simulink model "control"  (R2022a)
settings: Solver=FixedStepAuto  StartTime=0.0  StopTime=Inf  FixedStep=Ts  RelTol=1e-3  EnableMultiTasking=on
undefined symbols (not defined in the file): Analog_max, Calib_Gain, GPTRIP1SEL, Ipeak, Ki_i, Kp_i, Kp_w, Kt, Offset, Ts, TZ1, V_AImax, Vbat, Vnom, w_motor_max
libraries: c2837xDlib x3, c2802xlib x3, slpidlib x2, c280xlib x2
settings Model: SimulationMode=external  ExtModeTrigDuration=8  Creator=34688  LastModifiedBy=manu.sanchez
settings SolverCC: AutoInsertRateTranBlk=on
settings OptimizationCC: DefaultUnderspecifiedDataType=single  EnhancedBackFolding=on  PassReuseOutputArgsAs=Individual arguments  MaxStackSize=1024  OptimizeBlockOrder=speed  DifferentSizesBufferReuse=on  OptimizationCustomize=off  DenormalBehavior=FlushToZero  EfficientTunableParamExpr=on
settings DebuggingCC: ParameterTunabilityLossMsg=error  UnconnectedInputMsg=warning  UnconnectedOutputMsg=warning  UnconnectedLineMsg=warning
settings HardwareCC: ProdBitPerChar=16  ProdBitPerInt=16  ProdBitPerPointer=32  ProdBitPerSizeT=32  ProdBitPerPtrDiffT=32  ProdLargestAtomicInteger=Integer  ProdLargestAtomicFloat=None  ProdWordSize=16  ProdLongLongMode=on  ProdHWDeviceType=Texas Instruments->C2000
settings SFSimCC: MATLABDynamicMemAlloc=off
settings RTWCC: SystemTargetFile=ert.tlc  HardwareBoard=TI Delfino F28379D LaunchPad  TemplateMakefile=ert_default_tmf  Toolchain=Texas Instruments Code Composer Studio (C2000)  DLArmComputeVersion=19.05
settings CodeAppCC: ForceParamTrailComments=on  IgnoreCustomStorageClasses=off  OperatorAnnotations=on  SimulinkDataObjDesc=on  SFDataObjDesc=on  InsertBlockDesc=on
settings ERTTargetCC: CodeReplacementLibrary=TI C28x  SupportContinuousTime=on  ExtModeTransport=3  ExtModeStaticAllocSize=10000

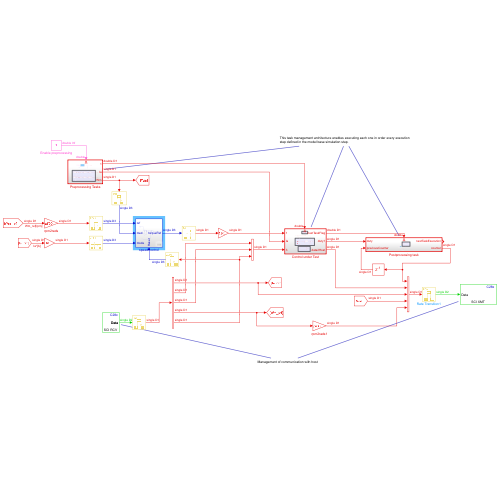
[thumbnail: Simulink's stored preview of the top-level diagram]
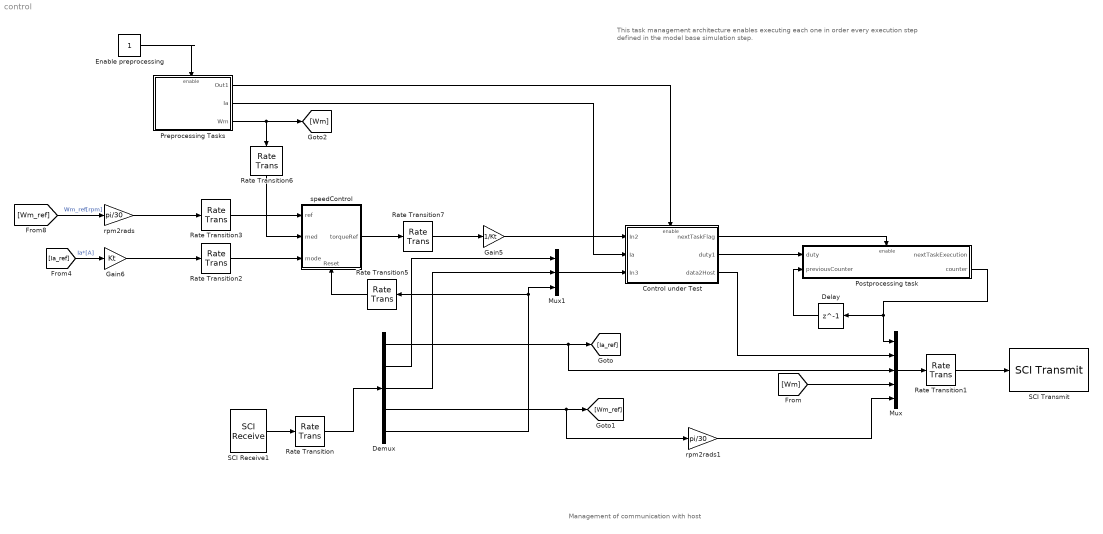
== system control ==
  note: This task management architecture enables executing each one in order every execution step defined in the model base simulation step.
  note: Management of communication with host
  Control under Test : Subsystem  TreatAsAtomicUnit=on
  Delay : Delay  DelayLength=1
  Demux : Demux  Outputs=5
  Enable preprocessing : Constant
  Gain5 : Gain  Gain=1/Kt
  Gain6 : Gain  Gain=Kt
  Mux : Mux  Inputs=5
  Mux1 : Mux  Inputs=3
  Postprocessing task : Subsystem  TreatAsAtomicUnit=on
  Preprocessing Tasks : Subsystem  TreatAsAtomicUnit=on
  Rate Transition : RateTransition  OutPortSampleTime=Ts
  Rate Transition1 : RateTransition  OutPortSampleTime=1e-3
  Rate Transition{2..3,5..6} (4 alike) : RateTransition  OutPortSampleTime=Ts*10
  Rate Transition7 : RateTransition  OutPortSampleTime=Ts
  SCI Receive1 : c280xlib/SCI Receive  sciModule=A  dataHead='S'  headerCheckMaxCount=16  dataTail='E'  dataType=single  dataLenOptions=Length via dialog  dataDim=5  maxDataLength=1  initValue=0  errOption=Output the last received value  errValue=0  sampleTime=0.001  blockingMode=on  timeOut=0.00875  outputStatus=off
      settings: SourceProductBaseCode=TIC2000
  SCI Transmit : c280xlib/SCI Transmit  sciModule=A  dataHead='S'  dataTail='E'  blockingMode=on  outputStatus=off
  rpm2rads : Gain  Gain=pi/30
  rpm2rads1 : Gain  Gain=pi/30
  speedControl : Subsystem
      settings: PortSchema="{\"entries\":[{\"content\":{\"sides\":[{\"content\":{\"connectorIds\":[\"In1\",\"In2\",\"In3\"]},\"type\":\"ConnectorPlacement.EquallySpacedRectSide\",\"uuid\":\"717e16ee-b0d7-408d-ae9c-739de9edb354\"},{\"content\":{\"connectorIds\":[\"Out1\"],\"side\":\"RIGHT\"},\"type\":\"ConnectorPlacement.EquallySpacedRectSide\",\"uuid\":\"4d51b045-d1f8-4970-b864-a989cb97e64e\"},{\"content\":{\"connectorIds\":[],\"side\":\"TOP\"},\"type\":\"ConnectorPlacement.EquallySpacedRectSide\",\"uuid\":\"4742e6f1-9767-49c3-9346-1403913518ce\"},{\"content\":{\"connectorIds\":[\"In4\"],\"side\":\"BOTTOM\"},\"type\":\"ConnectorPlacement.EquallySpacedRectSide\",\"uuid\":\"c526dc22-4687-4073-9922-de56cfbf6450\"}]},\"type\":\"ConnectorPlacement.EquallySpacedConnector\",\"uuid\":\"5f2e596d-c564-4cf7-8e3e-10d76f0f6b09\"}],\"packageUris\":[\"http://schema.mathworks.com/mf0/Connector/R2020b\"],\"version\":\"1.0\"}"
  wires:
  Control under Test/1(nextTaskFlag) -> Postprocessing task/Enable
  Enable preprocessing/1 -> Preprocessing Tasks/Enable
  SCI Receive1/1 -> Rate Transition/1
  Rate Transition1/1 -> SCI Transmit/1
  Control under Test/2(duty1) -> Postprocessing task/1(duty)
  Mux/1 -> Rate Transition1/1
  Control under Test/3(data2Host) -> Mux/2
  Postprocessing task/2(counter) -> Mux/1, Delay/1
  Delay/1 -> Postprocessing task/2(previousCounter)
  Preprocessing Tasks/1(Out1) -> Control under Test/Enable
  [Wm_ref] -> rpm2rads/1  "Wm_ref[rpm]"
  Gain6/1 -> Rate Transition2/1
  Preprocessing Tasks/3(Wm) -> Rate Transition6/1, [Wm]
  Demux/5 -> Rate Transition5/1, Mux1/3
  rpm2rads/1 -> Rate Transition3/1
  [Ia_ref] -> Gain6/1  "Ia*[A]"
  speedControl/1(torqueRef) -> Rate Transition7/1
  Rate Transition/1 -> Demux/1
  Demux/1 -> Mux/3, [Ia_ref]
  Demux/4 -> rpm2rads1/1, [Wm_ref]
  Mux1/1 -> Control under Test/3(In3)
  Demux/2 -> Mux1/1
  Demux/3 -> Mux1/2
  Preprocessing Tasks/2(Ia) -> Control under Test/2(Ia)
  Rate Transition2/1 -> speedControl/3(mode)
  Rate Transition3/1 -> speedControl/1(ref)
  Gain5/1 -> Control under Test/1(In2)
  Rate Transition5/1 -> speedControl/4(Reset)
  Rate Transition6/1 -> speedControl/2(med)
  Rate Transition7/1 -> Gain5/1
  [Wm] -> Mux/4
  rpm2rads1/1 -> Mux/5

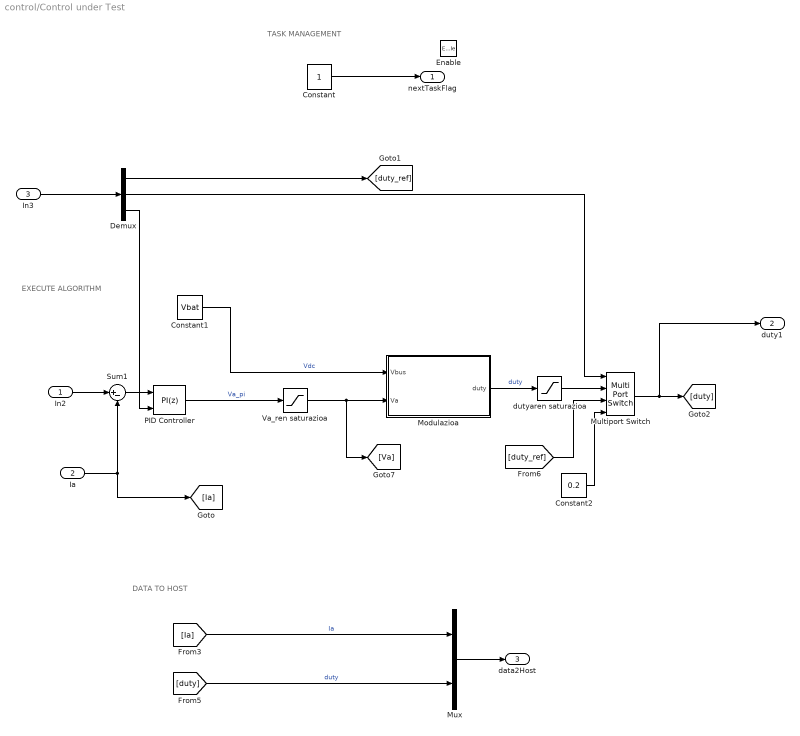
== system control/Control under Test ==
  note: TASK MANAGEMENT
  note: EXECUTE ALGORITHM
  note: DATA TO HOST
  In2 : Inport
  Ia : Inport  Port=2
  In3 : Inport  Port=3
  Enable : EnablePort
  Constant : Constant
  Constant1 : Constant  Value=Vbat  OutDataTypeStr=single
  Constant2 : Constant  Value=0.2  OutDataTypeStr=single  SampleTime=200e-6
  Demux : Demux  Outputs=3
  Modulazioa : Subsystem  Variant=on  VariantControlMode=label  LabelModeActiveChoice=MODULAZIOA_ZUBI_ERDIA  mask{LabelModeActiveChoice=MODULAZIOA_ZUBI_ERDIA}
      mask prompts: LabelModeActiveChoice "Simulink:Variants:LabelComboBox"
      mask TypeOptions LabelModeActiveChoice: LabelModeActiveChoice
      mask DialogControl LabelModeActiveChoice Prompt: Label mode active choice:
  Multiport Switch : MultiPortSwitch  SaturateOnIntegerOverflow=off  InputSameDT=off
  Mux : Mux  Inputs=2
  PID Controller : slpidlib/PID Controller  Controller=PI  Form=Parallel  TimeDomain=Discrete-time  UseExternalTs=off  SampleTime=Ts  IntegratorMethod=Forward Euler  FilterMethod=Forward Euler  ControllerParametersSource=internal  P=Kp_i  I=Ki_i  UseKiTs=off  D=0  N=100  UseFilter=on  TunerSelectOption=Transfer Function Based (PID Tuner App)  InitialConditionSource=internal  InitialConditionForIntegrator=0  InitialConditionForFilter=0  DifferentiatorICPrevScaledInput=0  ExternalReset=rising  TrackingMode=off  Kt=1  LimitOutput=on  SatLimitsSource=internal  UpperSaturationLimit=inf  LowerSaturationLimit=-inf  LinearizeAsGain=on  AntiWindupMode=back-calculation  Kb=1  POutMin=[]  POutMax=[]  IOutMin=[]  IOutMax=[]  DOutMin=[]  DOutMax=[]  NOutMin=[]  NOutMax=[]  SumOutMin=[]  SumOutMax=[]  SaturationOutMin=[]  SaturationOutMax=[]  PParamMin=[]  PParamMax=[]  IParamMin=[]  IParamMax=[]  DParamMin=[]  DParamMax=[]  NParamMin=[]  NParamMax=[]  KbParamMin=[]  KbParamMax=[]  KtParamMin=[]  KtParamMax=[]  KbOutMin=[]  KbOutMax=[]  KtOutMin=[]  KtOutMax=[]  IntegratorOutMin=[]  IntegratorOutMax=[]  FilterOutMin=[]  FilterOutMax=[]  SumI1OutMin=[]  SumI1OutMax=[]  SumI2OutMin=[]  SumI2OutMax=[]  SumI3OutMin=[]  SumI3OutMax=[]  SumI4OutMin=[]  SumI4OutMax=[]  SumDOutMin=[]  SumDOutMax=[]  DifferentiatorOutMin=[]  DifferentiatorOutMax=[]  FilterDiffOutCoefMin=[]  FilterDiffOutCoefMax=[]  ReciprocalOutMin=[]  ReciprocalOutMax=[]  SumDenOutMin=[]  SumDenOutMax=[]  SumNumOutMin=[]  SumNumOutMax=[]  DivideOutMin=[]  DivideOutMax=[]  UdiffTsProdOutMin=[]  UdiffTsProdOutMax=[]  NTsProdOutMin=[]  NTsProdOutMax=[]  UintegralTsProdOutMin=[]  UintegralTsProdOutMax=[]  UngainTsProdOutMin=[]  UngainTsProdOutMax=[]  IntegratorContinuousStateAttributes=''  IntegratorStateMustResolveToSignalObject=off  IntegratorRTWStateStorageClass=Auto  FilterContinuousStateAttributes=''  FilterStateMustResolveToSignalObject=off  FilterRTWStateStorageClass=Auto  ParallelPVariant=InternalParameters  IdealPVariant=Disabled  IVariant=InternalParameters  DVariant=Disabled  IntegratorVariant=Discrete  SatVariant=Enabled  AWVariant=BackCalculation  PCopyVariant=Disabled  TRVariant=Disabled  FdbkBlocksVariant=Forward  IdealPFdbkVariant=Disabled  SatFdbkVariant=Disabled  DerivativeFilterVariant=Disabled  NVariant=Disabled  NCopyVariant=Disabled_SignalSpec  FilterICVariant=Disabled  IntegratorICVariant=InternalICs  ExternalResetVariant=ExternalReset  TRSumVariant=Passthrough  SumFdbkVariant=Disabled  SumVariant=Sum_PI  TsampFilterVariant=InternalTs  TsampNgainVariant=Passthrough  TsampIntegralVariant=Passthrough  ExternalSaturationOutDataTypeStr=Inherit: Same as second input  aMode=0
  Sum1 : Sum  Inputs=|+-
  Va_ren saturazioa : Saturate  UpperLimit=Vnom  LowerLimit=0
  dutyaren saturazioa : Saturate  UpperLimit=1  LowerLimit=0
  nextTaskFlag : Outport
  duty1 : Outport  Port=2
  data2Host : Outport  Port=3
  wires:
  Constant/1 -> nextTaskFlag/1
  PID Controller/1 -> Va_ren saturazioa/1  "Va_pi"
  Modulazioa/1("duty ") -> dutyaren saturazioa/1  "duty"
  [duty] -> Mux/2  "duty"
  dutyaren saturazioa/1 -> Multiport Switch/2
  Constant2/1 -> Multiport Switch/4
  [duty_ref] -> Multiport Switch/3
  [Ia] -> Mux/1  "Ia"
  Va_ren saturazioa/1 -> Modulazioa/2(Va), [Va]
  Mux/1 -> data2Host/1
  Ia/1 -> Sum1/2, [Ia]
  Sum1/1 -> PID Controller/1
  Constant1/1 -> Modulazioa/1(Vbus)  "Vdc"
  Demux/3 -> PID Controller/2
  In2/1 -> Sum1/1
  In3/1 -> Demux/1
  Demux/1 -> [duty_ref]
  Demux/2 -> Multiport Switch/1
  Multiport Switch/1 -> duty1/1, [duty]

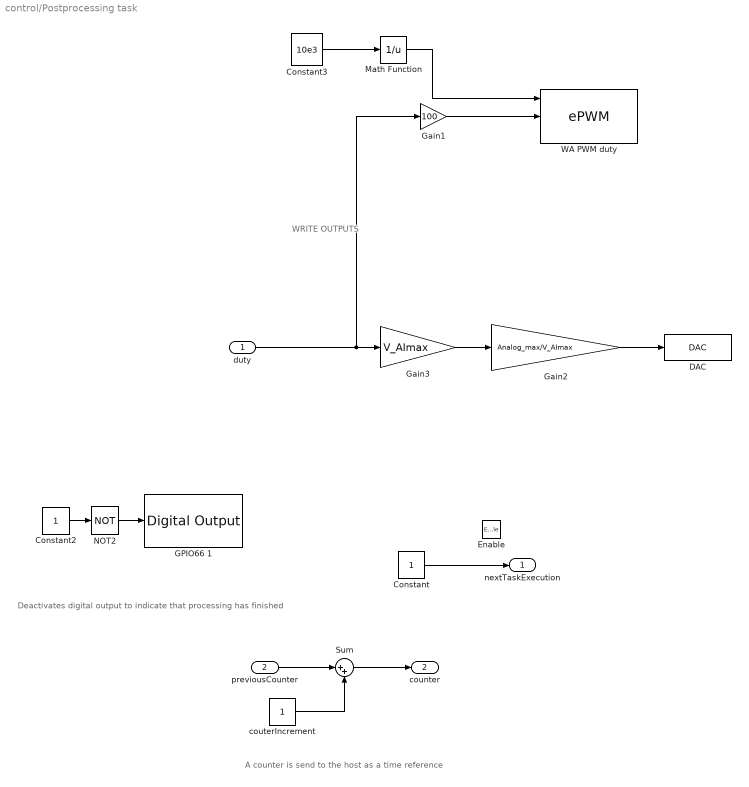
== system control/Postprocessing task ==
  note: A counter is send to the host as a time reference
  note: Deactivates digital output to indicate that processing has finished
  note: WRITE OUTPUTS
  duty : Inport
  previousCounter : Inport  Port=2
  Enable : EnablePort
  Constant : Constant
  Constant2 : Constant
  Constant3 : Constant  Value=10e3  OutDataTypeStr=single  SampleTime=200e-6
  DAC : c2837xDlib/DAC  channel=A  saturate=on
      settings: SourceProductBaseCode=TIC2000
  GPIO66 1 : c2837xDlib/Digital Output  GPIO_Number=GPIO0~GPIO7  GPIO_Bit0=on  GPIO_BIT0_Toggle=off  GPIO_Bit1=off  GPIO_BIT1_Toggle=off  GPIO_Bit2=off  GPIO_BIT2_Toggle=off  GPIO_Bit3=off  GPIO_BIT3_Toggle=off  GPIO_Bit4=off  GPIO_BIT4_Toggle=on  GPIO_Bit5=off  GPIO_BIT5_Toggle=on  GPIO_Bit6=off  GPIO_BIT6_Toggle=off  GPIO_Bit7=off  GPIO_BIT7_Toggle=off
      settings: SourceProductBaseCode=TIC2000
  Gain1 : Gain  Gain=100
  Gain2 : Gain  Gain=Analog_max/V_AImax
  Gain3 : Gain  Gain=V_AImax
  Math Function : Math  Operator=reciprocal
  NOT2 : Logic  Operator=NOT  IconShape=distinctive  AllPortsSameDT=off  OutDataTypeStr=boolean
  Sum : Sum  Inputs=|++
  WA PWM duty : c2802xlib/ePWM  PwmType=C2000_Type4  useModule=ePWM4  ePWMxLINKTBPRD=Not Linked  periodUnits=Seconds  timerSource=Input port  timerPeriod_clk=64000  timerPeriod_sec=1/10000  tbshadow=Counter equals to zero  countingMode=Up  phaseActiveEnable=Disable  phaseDirection=Count down after sync  phaseActive=0  synchronizationEnable=off  dcaevt1Sync=off  dcbevt1Sync=off  synchronizationOption=Disable  perSynchronizationOption=Counter equals to period (CTR=PRD)  clockPrescale=1  HSclockPrescale=1  enswap=off  ePWMxAStatus=on  ePWMxAactionLogic1=Set  ePWMxAactionLogic2=Clear  ePWMxAactionLogic3=Clear  ePWMxAactionLogic4=Set  ePWMxAactionLogic5=Do nothing  ePWMxAactionLogic6=Do nothing  ePWMxACSFenable=off  ePWMxACSFvalue=Forcing disable  ePWMxASFreload=Zero  ePWMxBStatus=off  ePWMxBactionLogic1=Set  ePWMxBactionLogic2=Clear  ePWMxBactionLogic3=Do nothing  ePWMxBactionLogic4=Do nothing  ePWMxBactionLogic5=Clear  ePWMxBactionLogic6=Set  ePWMxBCSFenable=off  ePWMxBCSFvalue=Forcing disable  ePWMxBSFreload=Zero  ePWNxBOutWay=off  ePWMxLINKCMPA=Not Linked  CMPAUnits=Percentages  CMPASource=Input port  CMPAValue_per=50  CMPAValue_clk=32000  enCMPAshadow=Counter equals to zero (CTR=Zero)  ePWMxLINKCMPB=Not Linked  CMPBUnits=Percentages  CMPBSource=Input port  CMPBValue_per=50  CMPBValue_clk=32000  enCMPBshadow=Counter equals to zero (CTR=Zero)  ePWMxLINKCMPC=Not Linked  CMPCUnits=Clock cycles  CMPCSource=Specify via dialog  CMPCValue_per=50  CMPCValue_clk=32000  enCMPCshadow=Counter equals to zero (CTR=Zero)  ePWMxLINKCMPD=Not Linked  CMPDUnits=Clock cycles  CMPDSource=Specify via dialog  CMPDValue_per=50  CMPDValue_clk=32000  enCMPDshadow=Counter equals to zero (CTR=Zero)  enableDBePWMxA=off  enableDBePWMxB=off  enhalfcycle=off  DBpolarity=Active high (AH)  DBedgeDelay=Positive  DBSource_ePWMxA=ePWMxA  DBSource_ePWMxB=ePWMxA  DBPeriodUnits=Clock cycles  DBperiodSource=Specify via dialog  REDperiod=0  FEDperiod=0  REDperiod_sec=0  FEDperiod_sec=0  LoadModeDBRED=Immediate without using shadow  LoadModeDBFED=Immediate without using shadow  adcstartModuleA=off  adcrequestEventA=First event  adcstartEventA=Digital Compare Module A Event 1 start of conversion (DCAEVT1.soc)  adcstartEventA_type2=Counter equals to zero (CTR=Zero)  adcstartModuleB=off  adcrequestEventB=First event  adcstartEventB=Counter equals to zero (CTR=Zero)  adcstartEventB_type2=Counter equals to zero (CTR=Zero)  intEn=off  intPrd=First event  intSel=Counter equals to zero (CTR=Zero)  intSel_type2=Counter equals to zero (CTR=Zero)  hrpe=off  enHRPWM=off  HRPWM_LoadMode=Counter equals to period (CTR=PRD)  HRPWM_CTLMode=Duty or Period control mode  HRPWM_EDGMode=Both edge  hrpeb=off  enHRPWMB=off  HRPWM_LoadModeB=Counter equals to zero (CTR=ZERO)  HRPWM_CTLModeB=Duty or Period control mode  HRPWM_EDGModeB=Both edge  enHRDBRED=off  enHRDBFED=off  enSFO=on  enautoconv=on  chopperEnable=off  chopperFrequency=1  chopperFirstwidth=1  chopperDuty=12.5%  tripZonesource=Specify via dialog  tzselOSHT1=off  tzselOSHT2=off  tzselOSHT3=off  tzselOSHDCAEV1=off  tzselOSHDCBEV1=off  tzselCBC1=off  tzselCBC2=off  tzselCBC3=off  tzselCBCDCAEV2=off  tzselCBCDCBEV2=off  tzselOSHT4=off  tzselOSHT5=off  tzselOSHT6=off  tzselCBC4=off  tzselCBC5=off  tzselCBC6=off  enTzOstIntr=off  enTzCbcIntr=off  enTzDCAEVT1Intr=off  enTzDCAEVT2Intr=off  enTzDCBEVT1Intr=off  enTzDCBEVT2Intr=off  ePWMxAforced=No action  ePWMxBforced=No action  DCAEVT1forced=No action  DCBEVT1forced=No action  DCAEVT2forced=No action  DCBEVT2forced=No action  dcah=Trip Zone 1 input (TZ1)  dcal=Trip Zone 2 input (TZ2)  dcbh=Trip Zone 1 input (TZ1)  dcbl=Trip Zone 2 input (TZ2)  dcah_type2=GPTRIP1SEL/(TZ1)  dcal_type2=GPTRIP1SEL/(TZ1)  dcbh_type2=GPTRIP1SEL/(TZ1)  dcbl_type2=GPTRIP1SEL/(TZ1)  gendcaevt1=Event disabled  gendcaevt2=Event disabled  gendcbevt1=Event disabled  gendcbevt2=Event disabled  dcaevt1src=DCAEVT1 with sync  dcaevt2src=DCAEVT2 with sync  dcbevt1src=DCBEVT1 with sync  dcbevt2src=DCBEVT2 with sync  pulsesel=Counter equals to zero (CTR=Zero)  blankinv=off  blankoffset=0  blankwidth=0  evsrcsel=Filtered version of DCAEVT1 (DCAEVT1FILT)  encape=off
  couterIncrement : Constant  OutDataTypeStr=single
  nextTaskExecution : Outport
  counter : Outport  Port=2
  wires:
  Constant/1 -> nextTaskExecution/1
  Constant2/1 -> NOT2/1
  NOT2/1 -> GPIO66 1/1
  previousCounter/1 -> Sum/1
  couterIncrement/1 -> Sum/2
  Sum/1 -> counter/1
  Gain2/1 -> DAC/1
  Gain3/1 -> Gain2/1
  Gain1/1 -> WA PWM duty/2
  Math Function/1 -> WA PWM duty/1
  duty/1 -> Gain1/1, Gain3/1
  Constant3/1 -> Math Function/1

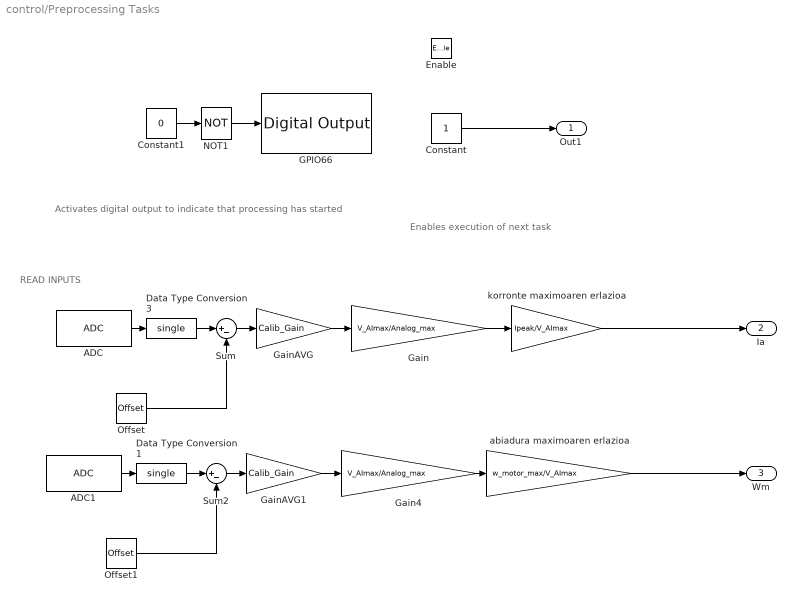
== system control/Preprocessing Tasks ==
  note: Enables execution of next task
  note: Activates digital output to indicate that processing has started
  note: READ INPUTS
  Enable : EnablePort
  ADC : c2802xlib/ADC  blkParamProc=C2000_Type4  ADCModule=A  samplingMode=Single sample mode  ADCResolution=12-bit (Single-ended input)  useSOC1=SOC0  useSOC2=SOC0_SOC1  SOCAcquisitionWindow=15  SOCTriggerSource=Software  SOCInterruptTrigger=No ADCINT  Ts=Ts  dType=uint16  postInterrupt=off  interruptSel=ADCINT1  ADCINTContinuous=on  endma=off  chdma=1  conv1=ADCINA0  conv2=ADCINA0 and ADCINB0  conv1_Type4=ADCIN15  conv2_Type4=ADCIN0 and ADCIN1
  ADC1 : c2802xlib/ADC  blkParamProc=C2000_Type4  ADCModule=B  samplingMode=Single sample mode  ADCResolution=12-bit (Single-ended input)  useSOC1=SOC0  useSOC2=SOC0_SOC1  SOCAcquisitionWindow=15  SOCTriggerSource=Software  SOCInterruptTrigger=No ADCINT  Ts=Ts  dType=uint16  postInterrupt=off  interruptSel=ADCINT1  ADCINTContinuous=on  endma=off  chdma=1  conv1=ADCINA0  conv2=ADCINA0 and ADCINB0  conv1_Type4=ADCIN5  conv2_Type4=ADCIN0 and ADCIN1
  Constant : Constant
  Constant1 : Constant  Value=0
  Data Type Conversion1 : DataTypeConversion  OutDataTypeStr=single  SaturateOnIntegerOverflow=off  RndMeth=Floor
  Data Type Conversion3 : DataTypeConversion  OutDataTypeStr=single  SaturateOnIntegerOverflow=off  RndMeth=Floor
  "GPIO66 " : c2837xDlib/Digital Output  GPIO_Number=GPIO0~GPIO7  GPIO_Bit0=on  GPIO_BIT0_Toggle=off  GPIO_Bit1=off  GPIO_BIT1_Toggle=off  GPIO_Bit2=off  GPIO_BIT2_Toggle=off  GPIO_Bit3=off  GPIO_BIT3_Toggle=off  GPIO_Bit4=off  GPIO_BIT4_Toggle=on  GPIO_Bit5=off  GPIO_BIT5_Toggle=on  GPIO_Bit6=off  GPIO_BIT6_Toggle=off  GPIO_Bit7=off  GPIO_BIT7_Toggle=off
      settings: SourceProductBaseCode=TIC2000
  Gain : Gain  Gain=V_AImax/Analog_max
  Gain4 : Gain  Gain=V_AImax/Analog_max
  GainAVG : Gain  Gain=Calib_Gain  OutDataTypeStr=single
  GainAVG1 : Gain  Gain=Calib_Gain  OutDataTypeStr=single
  NOT1 : Logic  Operator=NOT  IconShape=distinctive  AllPortsSameDT=off  OutDataTypeStr=boolean
  Offset : Constant  Value=Offset  OutDataTypeStr=single
  Offset1 : Constant  Value=Offset  OutDataTypeStr=single
  Sum : Sum  Inputs=|+-
  Sum2 : Sum  Inputs=|+-
  abiadura maximoaren erlazioa : Gain  Gain=w_motor_max/V_AImax
  korronte maximoaren erlazioa : Gain  Gain=Ipeak/V_AImax
  Out1 : Outport
  Ia : Outport  Port=2
  Wm : Outport  Port=3
  wires:
  Constant/1 -> Out1/1
  Constant1/1 -> NOT1/1
  NOT1/1 -> "GPIO66 "/1
  GainAVG/1 -> Gain/1
  Sum/1 -> GainAVG/1
  Data Type Conversion3/1 -> Sum/1
  Offset1/1 -> Sum2/2
  Gain4/1 -> abiadura maximoaren erlazioa/1
  Sum2/1 -> GainAVG1/1
  ADC1/1 -> Data Type Conversion1/1
  abiadura maximoaren erlazioa/1 -> Wm/1
  ADC/1 -> Data Type Conversion3/1
  korronte maximoaren erlazioa/1 -> Ia/1
  Offset/1 -> Sum/2
  Data Type Conversion1/1 -> Sum2/1
  GainAVG1/1 -> Gain4/1
  Gain/1 -> korronte maximoaren erlazioa/1

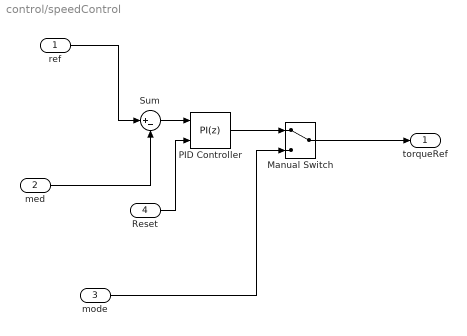
== system control/speedControl ==
  ref : Inport
  med : Inport  Port=2
  mode : Inport  Port=3
  Reset : Inport  Port=4
  Manual Switch : ManualSwitch
  PID Controller : slpidlib/PID Controller  Controller=PI  Form=Parallel  TimeDomain=Discrete-time  UseExternalTs=off  SampleTime=Ts*10  IntegratorMethod=Forward Euler  FilterMethod=Forward Euler  ControllerParametersSource=internal  P=Kp_w  I=0  UseKiTs=off  D=0  N=100  UseFilter=on  TunerSelectOption=Transfer Function Based (PID Tuner App)  InitialConditionSource=internal  InitialConditionForIntegrator=0  InitialConditionForFilter=0  DifferentiatorICPrevScaledInput=0  ExternalReset=rising  TrackingMode=off  Kt=1  LimitOutput=on  SatLimitsSource=internal  UpperSaturationLimit=inf  LowerSaturationLimit=-inf  LinearizeAsGain=on  AntiWindupMode=back-calculation  Kb=1  POutMin=[]  POutMax=[]  IOutMin=[]  IOutMax=[]  DOutMin=[]  DOutMax=[]  NOutMin=[]  NOutMax=[]  SumOutMin=[]  SumOutMax=[]  SaturationOutMin=[]  SaturationOutMax=[]  PParamMin=[]  PParamMax=[]  IParamMin=[]  IParamMax=[]  DParamMin=[]  DParamMax=[]  NParamMin=[]  NParamMax=[]  KbParamMin=[]  KbParamMax=[]  KtParamMin=[]  KtParamMax=[]  KbOutMin=[]  KbOutMax=[]  KtOutMin=[]  KtOutMax=[]  IntegratorOutMin=[]  IntegratorOutMax=[]  FilterOutMin=[]  FilterOutMax=[]  SumI1OutMin=[]  SumI1OutMax=[]  SumI2OutMin=[]  SumI2OutMax=[]  SumI3OutMin=[]  SumI3OutMax=[]  SumI4OutMin=[]  SumI4OutMax=[]  SumDOutMin=[]  SumDOutMax=[]  DifferentiatorOutMin=[]  DifferentiatorOutMax=[]  FilterDiffOutCoefMin=[]  FilterDiffOutCoefMax=[]  ReciprocalOutMin=[]  ReciprocalOutMax=[]  SumDenOutMin=[]  SumDenOutMax=[]  SumNumOutMin=[]  SumNumOutMax=[]  DivideOutMin=[]  DivideOutMax=[]  UdiffTsProdOutMin=[]  UdiffTsProdOutMax=[]  NTsProdOutMin=[]  NTsProdOutMax=[]  UintegralTsProdOutMin=[]  UintegralTsProdOutMax=[]  UngainTsProdOutMin=[]  UngainTsProdOutMax=[]  IntegratorContinuousStateAttributes=''  IntegratorStateMustResolveToSignalObject=off  IntegratorRTWStateStorageClass=Auto  FilterContinuousStateAttributes=''  FilterStateMustResolveToSignalObject=off  FilterRTWStateStorageClass=Auto  ParallelPVariant=InternalParameters  IdealPVariant=Disabled  IVariant=InternalParameters  DVariant=Disabled  IntegratorVariant=Discrete  SatVariant=Enabled  AWVariant=BackCalculation  PCopyVariant=Disabled  TRVariant=Disabled  FdbkBlocksVariant=Forward  IdealPFdbkVariant=Disabled  SatFdbkVariant=Disabled  DerivativeFilterVariant=Disabled  NVariant=Disabled  NCopyVariant=Disabled_SignalSpec  FilterICVariant=Disabled  IntegratorICVariant=InternalICs  ExternalResetVariant=ExternalReset  TRSumVariant=Passthrough  SumFdbkVariant=Disabled  SumVariant=Sum_PI  TsampFilterVariant=InternalTs  TsampNgainVariant=Passthrough  TsampIntegralVariant=Passthrough  ExternalSaturationOutDataTypeStr=Inherit: Same as second input  aMode=0
  Sum : Sum  Inputs=|+-
  torqueRef : Outport
  wires:
  PID Controller/1 -> Manual Switch/1
  ref/1 -> Sum/1
  Sum/1 -> PID Controller/1
  mode/1 -> Manual Switch/2
  Manual Switch/1 -> torqueRef/1
  med/1 -> Sum/2
  Reset/1 -> PID Controller/2

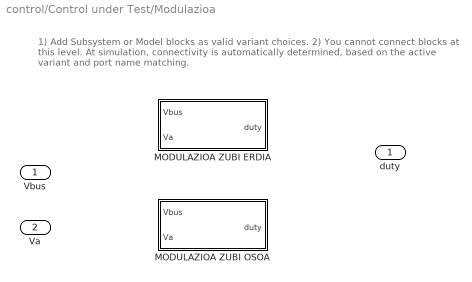
== system control/Control under Test/Modulazioa ==
  note: 1) Add Subsystem or Model blocks as valid variant choices.
      | 2) You cannot connect blocks at this level. At simulation, connectivity is automatically
      | determined, based on the active variant and port name matching.
  Vbus : Inport
  Va : Inport  Port=2
  MODULAZIOA ZUBI ERDIA : Subsystem  VariantControl=MODULAZIOA_ZUBI_ERDIA
  MODULAZIOA ZUBI OSOA : Subsystem  VariantControl=MODULAZIOA_ZUBI_OSOA
  "duty " : Outport

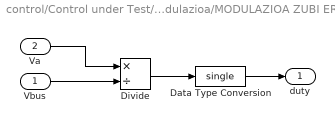
== system control/Control under Test/Modulazioa/MODULAZIOA ZUBI ERDIA ==
  Vbus : Inport
  Va : Inport  Port=2
  Data Type Conversion : DataTypeConversion  OutDataTypeStr=single  SaturateOnIntegerOverflow=off  RndMeth=Floor
  Divide : Product  Inputs=*/
  "duty " : Outport
  wires:
  Va/1 -> Divide/1
  Vbus/1 -> Divide/2
  Divide/1 -> Data Type Conversion/1
  Data Type Conversion/1 -> "duty "/1

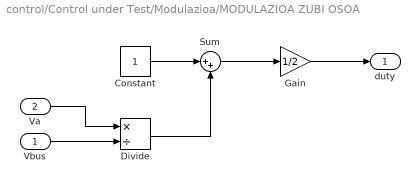
== system control/Control under Test/Modulazioa/MODULAZIOA ZUBI OSOA ==
  Vbus : Inport
  Va : Inport  Port=2
  Constant : Constant
  Divide : Product  Inputs=*/
  Gain : Gain  Gain=1/2
  Sum : Sum  Inputs=|++
  "duty " : Outport
  wires:
  Vbus/1 -> Divide/2
  Va/1 -> Divide/1
  Divide/1 -> Sum/2
  Constant/1 -> Sum/1
  Sum/1 -> Gain/1
  Gain/1 -> "duty "/1
